simulink model "Non_regulator_start"  (R2019b)
settings: Solver=VariableStepAuto  StartTime=0.0  StopTime=25  FixedStep=20e-3  MaxStep=20e-3  RelTol=1e-3
undefined symbols (not defined in the file): ang_output_relay, ang_switch_off_point, ang_switch_on_point, DiscIntNeverNeededParam, lin_output_relay, lin_switch_off_point, lin_switch_on_point, M
libraries: lib_robotinohardware x5, simulink x3
settings Model: EnablePacing=on  Creator=indorewala  LastModifiedBy=Олег
settings DataIOCC: LimitDataPoints=on  SaveFormat=Array  SignalLoggingSaveFormat=ModelDataLogs
settings OptimizationCC: ExpressionDepthLimit=2147483647  InitFltsAndDblsToZero=on  LifeSpan=inf
settings DebuggingCC: UnderspecifiedInitializationDetection=Classic  MergeDetectMultiDrivingBlocksExec=none  SolverPrmCheckMsg=warning  FcnCallInpInsideContextMsg=warning  StateNameClashWarn=warning  SFUnexpectedBacktrackingDiag=warning  SFNoUnconditionalDefaultTransitionDiag=warning  SFExecutionAtInitializationDiag=none  ArithmeticOperatorsInVariantConditions=warning
settings HardwareCC: ProdBitPerPointer=32  ProdBitPerSizeT=32  ProdBitPerPtrDiffT=32  ProdLargestAtomicFloat=None  ProdIntDivRoundTo=Undefined  ProdEndianess=Unspecified  ProdWordSize=32  ProdHWDeviceType=32-bit Generic
settings ModelReferenceCC: PropagateSignalLabelsOutOfModel=off
settings SFSimCC: SimUseLocalCustomCode=off  CustomCodeUndefinedFunction=UseInterfaceOnly
settings RTWCC: RTWUseLocalCustomCode=off
settings CodeAppCC: StateflowObjectComments=on
settings GRTTargetCC: TargetLangStandard=C89/C90 (ANSI)  CombineOutputUpdateFcns=off  GRTInterface=on
settings ConfigComp: CovMetricSettings=dw  CovHtmlReporting=on  CovSaveCumulativeToWorkspaceVar=on  CovSaveSingleToWorkspaceVar=on  CovExternalEMLEnable=off

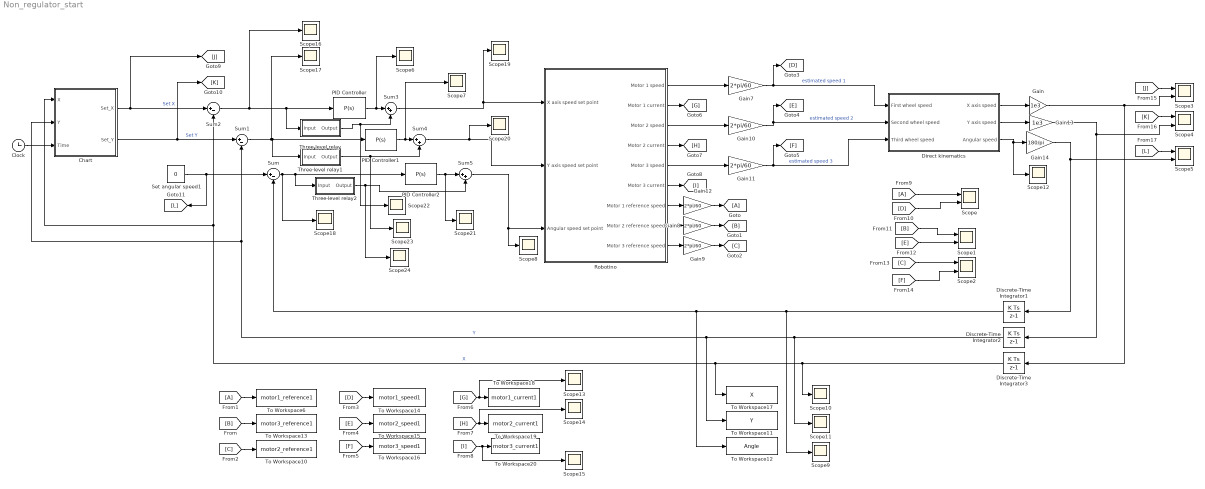
== system Non_regulator_start ==
  Chart : Stateflow chart  BlockKeywords=__PRM__SERIALIZED__DATA__:Stateflow Chart,Stateflow Diagram  TreatAsAtomicUnit=on
  Clock : Clock
  Direct kinematics : Subsystem
  Discrete-Time Integrator1 : DiscreteIntegrator  SampleTime=-1  ICPrevOutput=DiscIntNeverNeededParam  ICPrevScaledInput=DiscIntNeverNeededParam
  Discrete-Time Integrator2 : DiscreteIntegrator  SampleTime=-1  ICPrevOutput=DiscIntNeverNeededParam  ICPrevScaledInput=DiscIntNeverNeededParam
  Discrete-Time Integrator3 : DiscreteIntegrator  SampleTime=-1  ICPrevOutput=DiscIntNeverNeededParam  ICPrevScaledInput=DiscIntNeverNeededParam
  Gain : Gain  Gain=1e3
  Gain{7..12} (6 alike) : Gain  Gain=2*pi/60
  Gain13 : Gain  Gain=1e3
  Gain14 : Gain  Gain=180/pi
  PID Controller : simulink/Continuous/PID Controller  Controller=P  Form=Parallel  TimeDomain=Continuous-time  SampleTime=-1  IntegratorMethod=Forward Euler  FilterMethod=Forward Euler  ControllerParametersSource=internal  P=3  I=0.001  D=0  UseFilter=on  N=100  TunerSelectOption=Transfer Function Based (PID Tuner App)  InitialConditionSource=internal  InitialConditionForIntegrator=0  InitialConditionForFilter=0  DifferentiatorICPrevScaledInput=0  ExternalReset=none  TrackingMode=off  Kt=1  LimitOutput=on  UpperSaturationLimit=200  LowerSaturationLimit=-200  LinearizeAsGain=on  AntiWindupMode=none  Kb=1  POutMin=[]  POutMax=[]  IOutMin=[]  IOutMax=[]  DOutMin=[]  DOutMax=[]  NOutMin=[]  NOutMax=[]  SumOutMin=[]  SumOutMax=[]  SaturationOutMin=[]  SaturationOutMax=[]  PParamMin=[]  PParamMax=[]  IParamMin=[]  IParamMax=[]  DParamMin=[]  DParamMax=[]  NParamMin=[]  NParamMax=[]  KbParamMin=[]  KbParamMax=[]  KtParamMin=[]  KtParamMax=[]  KbOutMin=[]  KbOutMax=[]  KtOutMin=[]  KtOutMax=[]  IntegratorOutMin=[]  IntegratorOutMax=[]  FilterOutMin=[]  FilterOutMax=[]  SumI1OutMin=[]  SumI1OutMax=[]  SumI2OutMin=[]  SumI2OutMax=[]  SumI3OutMin=[]  SumI3OutMax=[]  SumI4OutMin=[]  SumI4OutMax=[]  SumDOutMin=[]  SumDOutMax=[]  DifferentiatorOutMin=[]  DifferentiatorOutMax=[]  FilterDiffOutCoefMin=[]  FilterDiffOutCoefMax=[]  ReciprocalOutMin=[]  ReciprocalOutMax=[]  SumDenOutMin=[]  SumDenOutMax=[]  SumNumOutMin=[]  SumNumOutMax=[]  DivideOutMin=[]  DivideOutMax=[]  IntegratorContinuousStateAttributes=''  IntegratorStateMustResolveToSignalObject=off  IntegratorRTWStateStorageClass=Auto  FilterContinuousStateAttributes=''  FilterStateMustResolveToSignalObject=off  FilterRTWStateStorageClass=Auto  ParallelPVariant=InternalParameters  IdealPVariant=Disabled  IVariant=Disabled  DVariant=Disabled  IntegratorVariant=Disabled  SatVariant=Enabled  AWVariant=Disabled  PCopyVariant=Disabled  TRVariant=Disabled  FdbkBlocksVariant=Forward  IdealPFdbkVariant=Disabled  SatFdbkVariant=Disabled  DerivativeFilterVariant=Disabled  NVariant=Disabled  NCopyVariant=Disabled_SignalSpec  FilterICVariant=Disabled  IntegratorICVariant=Disabled  ExternalResetVariant=Disabled  TRSumVariant=Passthrough  SumFdbkVariant=Disabled  SumVariant=Passthrough_P
  PID Controller1 : simulink/Continuous/PID Controller  Controller=P  Form=Parallel  TimeDomain=Continuous-time  SampleTime=-1  IntegratorMethod=Forward Euler  FilterMethod=Forward Euler  ControllerParametersSource=internal  P=3  I=0.001  D=0  UseFilter=on  N=100  TunerSelectOption=Transfer Function Based (PID Tuner App)  InitialConditionSource=internal  InitialConditionForIntegrator=0  InitialConditionForFilter=0  DifferentiatorICPrevScaledInput=0  ExternalReset=none  TrackingMode=off  Kt=1  LimitOutput=on  UpperSaturationLimit=200  LowerSaturationLimit=-200  LinearizeAsGain=on  AntiWindupMode=none  Kb=1  POutMin=[]  POutMax=[]  IOutMin=[]  IOutMax=[]  DOutMin=[]  DOutMax=[]  NOutMin=[]  NOutMax=[]  SumOutMin=[]  SumOutMax=[]  SaturationOutMin=[]  SaturationOutMax=[]  PParamMin=[]  PParamMax=[]  IParamMin=[]  IParamMax=[]  DParamMin=[]  DParamMax=[]  NParamMin=[]  NParamMax=[]  KbParamMin=[]  KbParamMax=[]  KtParamMin=[]  KtParamMax=[]  KbOutMin=[]  KbOutMax=[]  KtOutMin=[]  KtOutMax=[]  IntegratorOutMin=[]  IntegratorOutMax=[]  FilterOutMin=[]  FilterOutMax=[]  SumI1OutMin=[]  SumI1OutMax=[]  SumI2OutMin=[]  SumI2OutMax=[]  SumI3OutMin=[]  SumI3OutMax=[]  SumI4OutMin=[]  SumI4OutMax=[]  SumDOutMin=[]  SumDOutMax=[]  DifferentiatorOutMin=[]  DifferentiatorOutMax=[]  FilterDiffOutCoefMin=[]  FilterDiffOutCoefMax=[]  ReciprocalOutMin=[]  ReciprocalOutMax=[]  SumDenOutMin=[]  SumDenOutMax=[]  SumNumOutMin=[]  SumNumOutMax=[]  DivideOutMin=[]  DivideOutMax=[]  IntegratorContinuousStateAttributes=''  IntegratorStateMustResolveToSignalObject=off  IntegratorRTWStateStorageClass=Auto  FilterContinuousStateAttributes=''  FilterStateMustResolveToSignalObject=off  FilterRTWStateStorageClass=Auto  ParallelPVariant=InternalParameters  IdealPVariant=Disabled  IVariant=Disabled  DVariant=Disabled  IntegratorVariant=Disabled  SatVariant=Enabled  AWVariant=Disabled  PCopyVariant=Disabled  TRVariant=Disabled  FdbkBlocksVariant=Forward  IdealPFdbkVariant=Disabled  SatFdbkVariant=Disabled  DerivativeFilterVariant=Disabled  NVariant=Disabled  NCopyVariant=Disabled_SignalSpec  FilterICVariant=Disabled  IntegratorICVariant=Disabled  ExternalResetVariant=Disabled  TRSumVariant=Passthrough  SumFdbkVariant=Disabled  SumVariant=Passthrough_P
  PID Controller2 : simulink/Continuous/PID Controller  Controller=P  Form=Parallel  TimeDomain=Continuous-time  SampleTime=-1  IntegratorMethod=Forward Euler  FilterMethod=Forward Euler  ControllerParametersSource=internal  P=3  I=0.001  D=0  UseFilter=on  N=100  TunerSelectOption=Transfer Function Based (PID Tuner App)  InitialConditionSource=internal  InitialConditionForIntegrator=0  InitialConditionForFilter=0  DifferentiatorICPrevScaledInput=0  ExternalReset=none  TrackingMode=off  Kt=1  LimitOutput=on  UpperSaturationLimit=100  LowerSaturationLimit=-100  LinearizeAsGain=on  AntiWindupMode=none  Kb=1  POutMin=[]  POutMax=[]  IOutMin=[]  IOutMax=[]  DOutMin=[]  DOutMax=[]  NOutMin=[]  NOutMax=[]  SumOutMin=[]  SumOutMax=[]  SaturationOutMin=[]  SaturationOutMax=[]  PParamMin=[]  PParamMax=[]  IParamMin=[]  IParamMax=[]  DParamMin=[]  DParamMax=[]  NParamMin=[]  NParamMax=[]  KbParamMin=[]  KbParamMax=[]  KtParamMin=[]  KtParamMax=[]  KbOutMin=[]  KbOutMax=[]  KtOutMin=[]  KtOutMax=[]  IntegratorOutMin=[]  IntegratorOutMax=[]  FilterOutMin=[]  FilterOutMax=[]  SumI1OutMin=[]  SumI1OutMax=[]  SumI2OutMin=[]  SumI2OutMax=[]  SumI3OutMin=[]  SumI3OutMax=[]  SumI4OutMin=[]  SumI4OutMax=[]  SumDOutMin=[]  SumDOutMax=[]  DifferentiatorOutMin=[]  DifferentiatorOutMax=[]  FilterDiffOutCoefMin=[]  FilterDiffOutCoefMax=[]  ReciprocalOutMin=[]  ReciprocalOutMax=[]  SumDenOutMin=[]  SumDenOutMax=[]  SumNumOutMin=[]  SumNumOutMax=[]  DivideOutMin=[]  DivideOutMax=[]  IntegratorContinuousStateAttributes=''  IntegratorStateMustResolveToSignalObject=off  IntegratorRTWStateStorageClass=Auto  FilterContinuousStateAttributes=''  FilterStateMustResolveToSignalObject=off  FilterRTWStateStorageClass=Auto  ParallelPVariant=InternalParameters  IdealPVariant=Disabled  IVariant=Disabled  DVariant=Disabled  IntegratorVariant=Disabled  SatVariant=Enabled  AWVariant=Disabled  PCopyVariant=Disabled  TRVariant=Disabled  FdbkBlocksVariant=Forward  IdealPFdbkVariant=Disabled  SatFdbkVariant=Disabled  DerivativeFilterVariant=Disabled  NVariant=Disabled  NCopyVariant=Disabled_SignalSpec  FilterICVariant=Disabled  IntegratorICVariant=Disabled  ExternalResetVariant=Disabled  TRSumVariant=Passthrough  SumFdbkVariant=Disabled  SumVariant=Passthrough_P
  Robotino : Subsystem
  Scope{,1..5} (6 alike) : Scope  NumInputPorts=2
  Scope{6..24} (19 alike) : Scope
  Set angular speed1 : Constant  Value=0
  Sum : Sum  Inputs=|+-
  Sum1 : Sum  Inputs=|+-
  Sum2 : Sum  Inputs=|+-
  Sum3 : Sum  Inputs=|++
  Sum4 : Sum  Inputs=|++
  Sum5 : Sum  Inputs=|++
  Three-level relay : Subsystem
  Three-level relay1 : Subsystem
  Three-level relay2 : Subsystem
  To Workspace10 : ToWorkspace  VariableName=motor2_reference1  SaveFormat=Timeseries  SampleTime=-1
  To Workspace11 : ToWorkspace  VariableName=Y  SaveFormat=Timeseries  SampleTime=-1
  To Workspace12 : ToWorkspace  VariableName=Angle  SaveFormat=Timeseries  SampleTime=-1
  To Workspace13 : ToWorkspace  VariableName=motor3_reference1  SaveFormat=Timeseries  SampleTime=-1
  To Workspace14 : ToWorkspace  VariableName=motor1_speed1  SaveFormat=Timeseries  SampleTime=-1
  To Workspace15 : ToWorkspace  VariableName=motor2_speed1  SaveFormat=Timeseries  SampleTime=-1
  To Workspace16 : ToWorkspace  VariableName=motor3_speed1  SaveFormat=Timeseries  SampleTime=-1
  To Workspace17 : ToWorkspace  VariableName=X  SaveFormat=Timeseries  SampleTime=-1
  To Workspace18 : ToWorkspace  VariableName=motor1_current1  SaveFormat=Timeseries  SampleTime=-1
  To Workspace19 : ToWorkspace  VariableName=motor2_current1  SaveFormat=Timeseries  SampleTime=-1
  To Workspace20 : ToWorkspace  VariableName=motor3_current1  SaveFormat=Timeseries  SampleTime=-1
  To Workspace6 : ToWorkspace  VariableName=motor1_reference1  SaveFormat=Timeseries  SampleTime=-1
  wires:
  Gain14/1 -> Discrete-Time Integrator1/1, Scope5/2
  Direct kinematics/2(Y axis speed) -> Gain13/1
  Sum2/1 -> Scope16/1, Three-level relay/1(Input), PID Controller/1
  Robotino/7(Motor 1 reference speed) -> Gain12/1
  Gain12/1 -> [A]
  [L] -> Scope5/1
  Sum/1 -> Scope18/1, Three-level relay2/1(Input), PID Controller2/1
  Robotino/9(Motor 3 reference speed) -> Gain9/1
  Sum1/1 -> Scope17/1, Three-level relay1/1(Input), PID Controller1/1
  Robotino/8(Motor 2 reference speed) -> Gain8/1
  Robotino/3(Motor 2 speed) -> Gain10/1
  [I] -> Scope15/1, To Workspace20/1
  [C] -> To Workspace10/1
  Robotino/5(Motor 3 speed) -> Gain11/1
  [K] -> Scope4/1
  Discrete-Time Integrator3/1 -> Scope10/1, To Workspace17/1, Chart/1(X), Sum2/2  "X"
  Robotino/1(Motor 1 speed) -> Gain7/1
  Discrete-Time Integrator1/1 -> Sum/2, To Workspace12/1, Scope9/1
  Direct kinematics/1(X axis speed) -> Gain/1
  [F] -> Scope2/2
  Gain13/1 -> Discrete-Time Integrator2/1, Scope4/2
  [E] -> To Workspace15/1
  Robotino/4(Motor 2 current) -> [H]
  [E] -> Scope1/2
  [C] -> Scope2/1
  Direct kinematics/3(Angular speed) -> Scope12/1, Gain14/1
  [J] -> Scope3/1
  [H] -> Scope14/1, To Workspace19/1
  [A] -> To Workspace6/1
  [B] -> Scope1/1
  [G] -> Scope13/1, To Workspace18/1
  [A] -> Scope/1
  Gain7/1 -> [D], Direct kinematics/1("First wheel speed ")  "estimated speed 1"
  Gain8/1 -> [B]
  [F] -> To Workspace16/1
  [B] -> To Workspace13/1
  Set angular speed1/1 -> [L], Sum/1
  Gain10/1 -> [E], Direct kinematics/2("Second wheel speed ")  "estimated speed 2"
  Robotino/6(Motor 3 current) -> [I]
  Discrete-Time Integrator2/1 -> To Workspace11/1, Chart/2(Y), Sum1/2, Scope11/1  "Y"
  Gain9/1 -> [C]
  Robotino/2(Motor 1 current) -> [G]
  [D] -> Scope/2
  [D] -> To Workspace14/1
  Gain11/1 -> Direct kinematics/3("Third wheel speed "), [F]  "estimated speed 3"
  Gain/1 -> Discrete-Time Integrator3/1, Scope3/2
  PID Controller/1 -> Scope6/1, Sum3/1
  Three-level relay/1(Output) -> Scope22/1, Sum3/2
  Sum3/1 -> Scope19/1, Robotino/1(X axis speed set point)
  PID Controller1/1 -> Scope7/1, Sum4/1
  Three-level relay1/1(Output) -> Scope23/1, Sum4/2
  Sum4/1 -> Scope20/1, Robotino/2(Y axis speed set point)
  PID Controller2/1 -> Scope21/1, Sum5/1
  Three-level relay2/1(Output) -> Scope24/1, Sum5/2
  Sum5/1 -> Scope8/1, Robotino/3(Angular speed set point)
  Chart/1(Set_X) -> [J], Sum2/1  "Set X"
  Chart/2(Set_Y) -> [K], Sum1/1  "Set Y"
  Clock/1 -> Chart/3(Time)

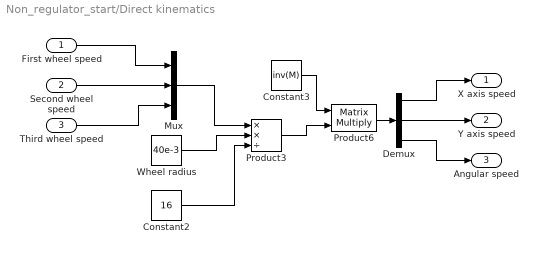
== system Non_regulator_start/Direct kinematics ==
  "First wheel speed " : Inport
  "Second wheel speed " : Inport  Port=2
  "Third wheel speed " : Inport  Port=3
  Constant2 : Constant  Value=16
  Constant3 : Constant  Value=inv(M)
  Demux : Demux  Outputs=3
  Mux : Mux  Inputs=3
  Product3 : Product  Inputs=**/
  Product6 : Product  Multiplication=Matrix(*)
  Wheel radius : Constant  Value=40e-3
  X axis speed : Outport
  Y axis speed : Outport  Port=2
  Angular speed : Outport  Port=3
  wires:
  Demux/2 -> Y axis speed/1
  Product6/1 -> Demux/1
  Constant3/1 -> Product6/1
  Demux/1 -> X axis speed/1
  Demux/3 -> Angular speed/1
  "Second wheel speed "/1 -> Mux/2
  "First wheel speed "/1 -> Mux/1
  "Third wheel speed "/1 -> Mux/3
  Mux/1 -> Product3/1
  Product3/1 -> Product6/2
  Wheel radius/1 -> Product3/2
  Constant2/1 -> Product3/3

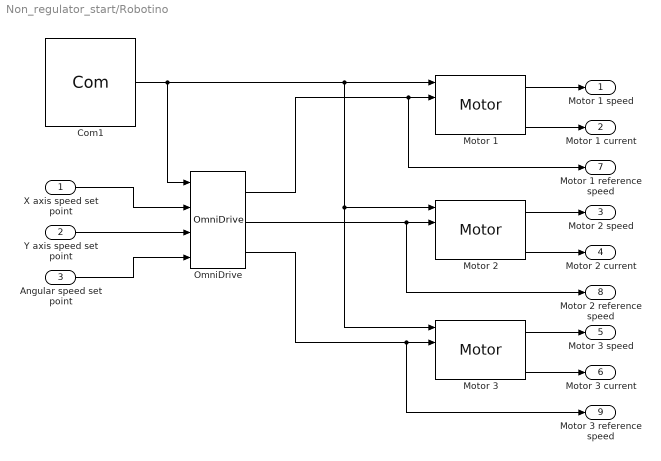
== system Non_regulator_start/Robotino ==
  X axis speed set point : Inport
  Y axis speed set point : Inport  Port=2
  Angular speed set point : Inport  Port=3
  Com1 : lib_robotinohardware/Com  ip='172.26.1.0'
  Motor 1 : lib_robotinohardware/Motor  num=0  kp=200  ki=10  kd=0
  Motor 2 : lib_robotinohardware/Motor  num=1  kp=200  ki=10  kd=0
  Motor 3 : lib_robotinohardware/Motor  num=2  kp=200  ki=10  kd=0
  OmniDrive : lib_robotinohardware/OmniDrive
  Motor 1 speed : Outport
  Motor 1 current : Outport  Port=2
  Motor 2 speed : Outport  Port=3
  Motor 2 current : Outport  Port=4
  Motor 3 speed : Outport  Port=5
  Motor 3 current : Outport  Port=6
  Motor 1 reference speed : Outport  Port=7
  Motor 2 reference speed : Outport  Port=8
  Motor 3 reference speed : Outport  Port=9
  wires:
  OmniDrive/2 -> Motor 2 reference speed/1, Motor 2/2
  OmniDrive/1 -> Motor 1 reference speed/1, Motor 1/2
  Com1/1 -> OmniDrive/1, Motor 1/1, Motor 3/1, Motor 2/1
  Angular speed set point/1 -> OmniDrive/4
  Motor 3/3 -> Motor 3 current/1
  OmniDrive/3 -> Motor 3 reference speed/1, Motor 3/2
  Motor 2/1 -> Motor 2 speed/1
  Motor 3/1 -> Motor 3 speed/1
  Motor 1/1 -> Motor 1 speed/1
  Motor 2/3 -> Motor 2 current/1
  X axis speed set point/1 -> OmniDrive/2
  Motor 1/3 -> Motor 1 current/1
  Y axis speed set point/1 -> OmniDrive/3

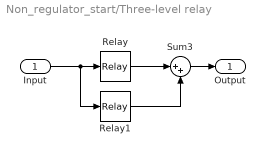
== system Non_regulator_start/Three-level relay ==
  Input : Inport
  Relay : Relay  OnSwitchValue=lin_switch_on_point  OffSwitchValue=lin_switch_off_point  OnOutputValue=lin_output_relay
  Relay1 : Relay  OnSwitchValue=-lin_switch_off_point  OffSwitchValue=-lin_switch_on_point  OnOutputValue=0  OffOutputValue=-lin_output_relay
  Sum3 : Sum  Inputs=|++
  Output : Outport
  wires:
  Input/1 -> Relay1/1, Relay/1
  Relay1/1 -> Sum3/2
  Relay/1 -> Sum3/1
  Sum3/1 -> Output/1

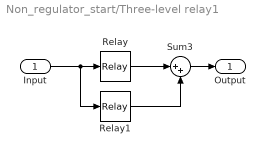
== system Non_regulator_start/Three-level relay1 ==
  Input : Inport
  Relay : Relay  OnSwitchValue=lin_switch_on_point  OffSwitchValue=lin_switch_off_point  OnOutputValue=lin_output_relay
  Relay1 : Relay  OnSwitchValue=-lin_switch_off_point  OffSwitchValue=-lin_switch_on_point  OnOutputValue=0  OffOutputValue=-lin_output_relay
  Sum3 : Sum  Inputs=|++
  Output : Outport
  wires:
  Sum3/1 -> Output/1
  Relay/1 -> Sum3/1
  Relay1/1 -> Sum3/2
  Input/1 -> Relay/1, Relay1/1

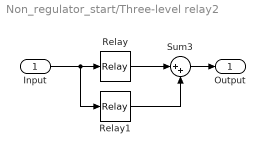
== system Non_regulator_start/Three-level relay2 ==
  Input : Inport
  Relay : Relay  OnSwitchValue=ang_switch_on_point  OffSwitchValue=ang_switch_off_point  OnOutputValue=ang_output_relay
  Relay1 : Relay  OnSwitchValue=-ang_switch_off_point  OffSwitchValue=-ang_switch_on_point  OnOutputValue=0  OffOutputValue=-ang_output_relay
  Sum3 : Sum  Inputs=|++
  Output : Outport
  wires:
  Input/1 -> Relay1/1, Relay/1
  Relay1/1 -> Sum3/2
  Relay/1 -> Sum3/1
  Sum3/1 -> Output/1

== stateflow chart Non_regulator_start/Chart ==
  state Forward
    during:
    Set_X = 1400;
    Set_Y = 0;
  state Stop
    during:
    Set_X = 0;
    Set_Y = 0;
  state Right
    during:
    Set_X = 0;
    Set_Y = 0;
  state Stop1
    entry:
    stop_time = Time;
    during:
    Set_X = 1400;
    Set_Y = 0;
  state Stop3
    entry:
    stop_time = Time;
    during:
    Set_X = 0;
    Set_Y = -400;
  state Stop2
    entry:
    stop_time = Time;
    during:
    Set_X = 1400;
    Set_Y = -400;
  state Left
    during:
    Set_X = 1400;
    Set_Y = -400;
  state Backward
    during:
    Set_X = 0;
    Set_Y = -400
  (default) -> Forward
  Right -> Stop : [Y>=0]
  Forward -> Stop1 : [X>=1400]
  Stop3 -> Right : [(Time - stop_time) > 0.2]
  Stop1 -> Left : [(Time - stop_time) > 0.2]
  Backward -> Stop3 : [X <= 0]
  Left -> Stop2 : [Y <= -400]
  Stop2 -> Backward : [(Time - stop_time) > 0.2]
  data: X input; Y input; Set_X output; Set_Y output; Time input; stop_time local
